simulink model "rocketSim"  (R2020a)
settings: Solver=ode3  StartTime=0.0  StopTime=9.9695  FixedStep=smp.h  MaxStep=simPrm.h  RelTol=1e-3
undefined symbols (not defined in the file): pln, rkt, thr
libraries: sm_lib x6, nesl_utility x6, simulink_extras x2
settings Model: Creator=ggparker  LastModifiedBy=crs20
settings SolverCC: NumberNewtonIterations=4
settings DataIOCC: ReturnWorkspaceOutputs=off  SignalLoggingName=rStates
settings DebuggingCC: PregeneratedLibrarySubsystemCodeDiagnostic=none  ArithmeticOperatorsInVariantConditions=warning
settings SFSimCC: SimUseLocalCustomCode=off  CustomCodeUndefinedFunction=UseInterfaceOnly
settings RTWCC: RTWUseLocalCustomCode=off
settings ExplorerConfigSet: InternalSimMechanicsExplorerSettings="<ExplorerConfiguration><canonicalview>planar_xy</canonicalview><AnimationSetting><BasePlaybackSpeed>1.0</BasePlaybackSpeed><PlaybackSpeedFactor>1.0</PlaybackSpeedFactor></AnimationSetting><TilePanel><TileInfo><Tiles Columns=\"1\" Count=\"1\" Rows=\"1\"><Column Weight=\"1\"/><Row Weight=\"1\"/><Tile Height=\"1\" Width=\"1\" X=\"0\" Y=\"0\"/></Tiles></TileInfo><SceneInfo><SceneViewer><BGColor><R>0.60000002384185791</R><G>0.60000002384185791</G><B>0.60000002384185791</B></BGColor><Camera><DoPerspective>off</DoPerspective><Position><X>282.141547094974555</X><Y>-19.3928666167923893</Y><Z>193.684626557609761</Z></Position><Center><X>282.141547094974555</X><Y>-19.3928666167923893</Y><Z>7.11250308427224809e-07</Z></Center><Up><X>0</X><Y>1</Y><Z>0</Z></Up><ViewLimDist>1</ViewLimDist><YLim>366.074836651506018</YLim><XLim>486.611673109928745</XLim></Camera></SceneViewer></SceneInfo></TilePanel><MechEditorPanel><Cameras/><GfxPanelCameraMap/><VideoCreator><PlaybackSpeedRatio>1.0</PlaybackSpeedRatio><FrameRate>30</FrameRate><VideoFormat>Motion JPEG AVI</VideoFormat><FrameSize>auto</FrameSize></VideoCreator></MechEditorPanel></ExplorerConfiguration>"

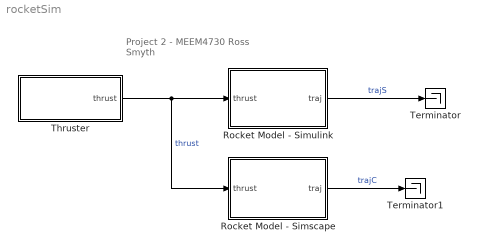
== system rocketSim ==
  note: Project 2 - MEEM4730
      | Ross Smyth
  Rocket Model - Simscape : Subsystem
  Rocket Model - Simulink : Subsystem
  Terminator : Terminator
  Terminator1 : Terminator
  Thruster : Subsystem
  wires:
  Rocket Model - Simulink/1(traj) -> Terminator/1  "trajS"
  Rocket Model - Simscape/1(traj) -> Terminator1/1  "trajC"
  Thruster/1(thrust) -> Rocket Model - Simscape/1(thrust), Rocket Model - Simulink/1(thrust)  "thrust"

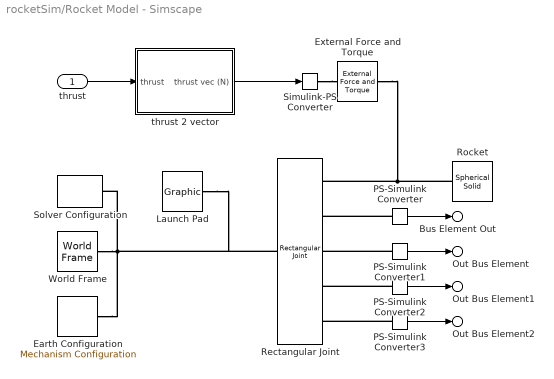
== system rocketSim/Rocket Model - Simscape ==
  thrust : Inport
  Earth Configuration : sm_lib/Utilities/Mechanism Configuration  UniformGravity=Constant  GravityVector=[0 -pln.g 0]  GravityUnits=m/s^2  LinearizationDelta=0.001
  External Force and Torque : sm_lib/Forces and Torques/External Force and Torque  ForceResolutionFrame=AttachedFrame  EnableForceX=off  EnableForceY=off  EnableForceZ=off  EnableForce=on  TorqueResolutionFrame=AttachedFrame  EnableTorqueX=off  EnableTorqueY=off  EnableTorqueZ=off  EnableTorque=off
  Launch Pad : sm_lib/Body Elements/Graphic  GraphicType=Marker  MarkerShape=Cube  MarkerSize=10  GraphicVisPropType=SimpleVisualProperties  GraphicDiffuseColor=[1.0 0.0 0.4]  GraphicSpecularColor=[0.5 0.5 0.5 1.0]  GraphicAmbientColor=[0.15 0.15 0.15 1.0]  GraphicEmissiveColor=[0.0 0.0 0.0 1.0]  GraphicShininess=75  GraphicOpacity=1.0
  PS-Simulink Converter{,1..3} (4 alike) : nesl_utility/PS-Simulink Converter  PhysicalDomain=network_engine_domain  SubClassName=ps_output  LeftPortType=input  RightPortType=output  PseudoPeriodic=off  Frequencies=[]  Unit=inherit  AffineConversion=off
  Rectangular Joint : sm_lib/Joints/Rectangular Joint  JointMode=Normal  SenseConstraintForce=off  SenseConstraintForceX=off  SenseConstraintForceY=off  SenseConstraintForceZ=off  SenseConstraintTorque=off  SenseConstraintTorqueX=off  SenseConstraintTorqueY=off  SenseConstraintTorqueZ=off  SenseTotalForce=off  SenseTotalForceX=off  SenseTotalForceY=off  SenseTotalForceZ=off  SenseTotalTorque=off  SenseTotalTorqueX=off  SenseTotalTorqueY=off  SenseTotalTorqueZ=off  CompositeWrenchDir=FollowerOnBase  CompositeWrenchFrame=BaseFrame  PxEquilibriumPosition=0  PxEquilibriumPositionUnits=m  PxSpringStiffness=0  PxSpringStiffnessUnits=N/m  PxDampingCoefficient=0  PxDampingCoefficientUnits=N/(m/s)  PxTorqueActuationMode=NoTorque  PxMotionActuationMode=ComputedMotion  PxSensePosition=on  PxSenseVelocity=on  PxSenseAcceleration=off  PxSenseTorqueForce=off  PxSenseLowerLimitTorqueForce=off  PxSenseUpperLimitTorqueForce=off  PxLowerLimitSpecify=off  PxLowerLimitBound=0  PxLowerLimitBoundUnits=m  PxLowerLimitStiffness=0  PxLowerLimitStiffnessUnits=N/m  PxLowerLimitDamping=0  PxLowerLimitDampingUnits=N/(m/s)  PxLowerLimitTransitionRegionWidth=0  PxLowerLimitTransitionRegionWidthUnits=m  PxUpperLimitSpecify=off  PxUpperLimitBound=1  PxUpperLimitBoundUnits=m  PxUpperLimitStiffness=1e6  PxUpperLimitStiffnessUnits=N/m  PxUpperLimitDamping=1e3  PxUpperLimitDampingUnits=N/(m/s)  PxUpperLimitTransitionRegionWidth=1e-4  PxUpperLimitTransitionRegionWidthUnits=m  PxPositionTargetSpecify=off  PxPositionTargetPriority=High  PxPositionTargetValue=0  PxPositionTargetValueUnits=m  PxVelocityTargetSpecify=off  PxVelocityTargetPriority=High  PxVelocityTargetValue=0  PxVelocityTargetValueUnits=m/s  PyEquilibriumPosition=0  PyEquilibriumPositionUnits=m  PySpringStiffness=0  PySpringStiffnessUnits=N/m  PyDampingCoefficient=0  PyDampingCoefficientUnits=N/(m/s)  PyTorqueActuationMode=NoTorque  PyMotionActuationMode=ComputedMotion  PySensePosition=on  PySenseVelocity=on  PySenseAcceleration=off  PySenseTorqueForce=off  PySenseLowerLimitTorqueForce=off  PySenseUpperLimitTorqueForce=off  PyLowerLimitSpecify=off  PyLowerLimitBound=-1  PyLowerLimitBoundUnits=m  PyLowerLimitStiffness=1e6  PyLowerLimitStiffnessUnits=N/m  PyLowerLimitDamping=1e3  PyLowerLimitDampingUnits=N/(m/s)  PyLowerLimitTransitionRegionWidth=1e-4  PyLowerLimitTransitionRegionWidthUnits=m  PyUpperLimitSpecify=off  PyUpperLimitBound=1  PyUpperLimitBoundUnits=m  PyUpperLimitStiffness=1e6  PyUpperLimitStiffnessUnits=N/m  PyUpperLimitDamping=1e3  PyUpperLimitDampingUnits=N/(m/s)  PyUpperLimitTransitionRegionWidth=1e-4  PyUpperLimitTransitionRegionWidthUnits=m  PyPositionTargetSpecify=off  PyPositionTargetPriority=High  PyPositionTargetValue=0  PyPositionTargetValueUnits=m  PyVelocityTargetSpecify=off  PyVelocityTargetPriority=High  PyVelocityTargetValue=0  PyVelocityTargetValueUnits=m/s
  Rocket : sm_lib/Body Elements/Spherical Solid  GraphicAmbientColor=[0.15 0.15 0.15 1.0]  BasedOnType=Mass  CenterOfMass=[0 0 0]  CenterOfMassUnits=m  GraphicDiffuseColor=[0.5 0.5 0.5]  Density=rkt.m  DensityUnits=kg/m^3  DoExposeReferenceFrame=on  GraphicEmissiveColor=[0.0 0.0 0.0 1.0]  ExportEntireGeometry=off  SerializedExposedGeometries=<ExposedGeometries/>  SerializedFrames=<Frames/>  MarkerShape=Sphere  MarkerSize=10  GraphicType=FromGeometry  InertiaType=PointMass  Mass=rkt.m  MassUnits=kg  MomentsOfInertia=[1 1 1]  MomentsOfInertiaUnits=kg*m^2  GraphicOpacity=1.0  ProductsOfInertia=[0 0 0]  ProductsOfInertiaUnits=kg*m^2  GraphicShininess=75  GraphicSpecularColor=[0.5 0.5 0.5 1.0]  SphereRadius=1  SphereRadiusUnits=m  GraphicVisPropType=SimpleVisualProperties
  Simulink-PS Converter : nesl_utility/Simulink-PS Converter  PhysicalDomain=network_engine_domain  SubClassName=ps_input  LeftPortType=input  RightPortType=output  PseudoPeriodic=off  Frequencies=[]  NoiseDistribution=none  NoiseParameters=[]  Unit=1  AffineConversion=off  FilteringAndDerivatives=provide  SimscapeFilterOrder=1  InputFilterTimeConstant=0.001  UdotUserProvided=0
  Solver Configuration : nesl_utility/Solver Configuration  PhysicalDomain=network_engine_domain  SubClassName=solver  LeftPortType=input  RightPortType=generic  Tones=[]  Harmonics=[]  SimulateNoise=off  Profile=off  UseLocalSampling=off  EnableSwitchedLinearOptims=on  FrequencyDomain=off  UseCCode=off  RelTol=0.001  AbsTol=1e-06  MinStep=1e-09  ToWorkspace=off  RevertToSquareIcSolve=off  NumHomotopyIterations=100  PhasorMode=off  PhasorModeNumHarmonics=1  DoDC=off  ResidualTolerance=1e-09  UseLocalSolver=off  LocalSolverChoice=NE_BACKWARD_EULER_ADVANCER  LocalSolverSampleTime=0.001  DoFixedCost=off  MaxNonlinIter=3  MaxModeIter=2  LinearAlgebra=auto  EquationFormulation=NE_TIME_EF  DelaysMemoryBudget=1024  AutomaticFiltering=on  FilteringTimeConstant=0.001  PartitionStorageMethod=AS_NEEDED  PartitionMemoryBudget=1024  PartitionMethod=ROBUST
  World Frame : sm_lib/Frames and Transforms/World Frame
  thrust 2 vector : Subsystem
  Bus Element Out : Outport  PortName=traj  Element=x
  Out Bus Element : Outport  PortName=traj  Element=xd
  Out Bus Element1 : Outport  PortName=traj  Element=y
  Out Bus Element2 : Outport  PortName=traj  Element=yd
  wires:
  thrust/1 -> thrust 2 vector/1(thrust)
  thrust 2 vector/1(thrust vec (N)) -> Simulink-PS Converter/1
  PS-Simulink Converter/1 -> Bus Element Out/1
  PS-Simulink Converter1/1 -> Out Bus Element/1
  PS-Simulink Converter2/1 -> Out Bus Element1/1
  PS-Simulink Converter3/1 -> Out Bus Element2/1
  connections:
  World Frame/RConn1 -- Launch Pad/RConn1 -- Rectangular Joint/LConn1 -- Solver Configuration/RConn1 -- Earth Configuration/RConn1
  PS-Simulink Converter/LConn1 -- Rectangular Joint/RConn2
  PS-Simulink Converter1/LConn1 -- Rectangular Joint/RConn3
  PS-Simulink Converter2/LConn1 -- Rectangular Joint/RConn4
  PS-Simulink Converter3/LConn1 -- Rectangular Joint/RConn5
  Simulink-PS Converter/RConn1 -- External Force and Torque/LConn1
  Rocket/RConn1 -- External Force and Torque/RConn1 -- Rectangular Joint/RConn1

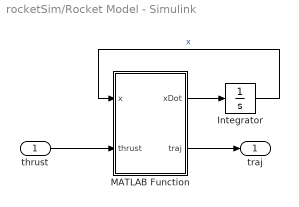
== system rocketSim/Rocket Model - Simulink ==
  thrust : Inport  OutDataTypeStr=Bus: thrust
  Integrator : Integrator  InitialCondition=rkt.ics
  MATLAB Function : MATLAB Function  TreatAsAtomicUnit=on
  traj : Outport  OutDataTypeStr=Bus: traj  VectorParamsAs1DForOutWhenUnconnected=off
  wires:
  MATLAB Function/2(traj) -> traj/1
  thrust/1 -> MATLAB Function/2(thrust)
  MATLAB Function/1(xDot) -> Integrator/1
  Integrator/1 -> MATLAB Function/1(x)  "x"

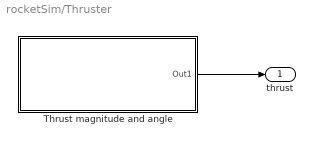
== system rocketSim/Thruster ==
  "Thrust magnitude and angle " : Subsystem  Variant=on  VariantControl=Choice
  thrust : Outport  OutDataTypeStr=Bus: thrust  VectorParamsAs1DForOutWhenUnconnected=off
  wires:
  "Thrust magnitude and angle "/1(Out1) -> thrust/1

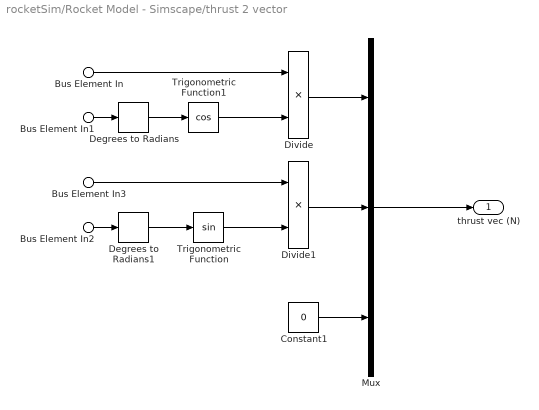
== system rocketSim/Rocket Model - Simscape/thrust 2 vector ==
  Bus Element In : Inport  PortName=thrust  Element=mag
  Bus Element In3 : Inport  PortName=thrust  Element=mag
  Bus Element In1 : Inport  PortName=thrust  Element=ang
  Bus Element In2 : Inport  PortName=thrust  Element=ang
  Constant1 : Constant  Value=0
  Degrees to Radians : simulink_extras/Transformations/Degrees to Radians
  Degrees to Radians1 : simulink_extras/Transformations/Degrees to Radians
  Divide : Product  Inputs=**
  Divide1 : Product  Inputs=**
  Mux : Mux  Inputs=3
  Trigonometric Function : Trigonometry
  Trigonometric Function1 : Trigonometry  Operator=cos
  thrust vec (N) : Outport  VectorParamsAs1DForOutWhenUnconnected=off
  wires:
  Trigonometric Function/1 -> Divide1/2
  Trigonometric Function1/1 -> Divide/2
  Degrees to Radians/1 -> Trigonometric Function1/1
  Bus Element In/1 -> Divide/1
  Bus Element In1/1 -> Degrees to Radians/1
  Bus Element In2/1 -> Degrees to Radians1/1
  Degrees to Radians1/1 -> Trigonometric Function/1
  Bus Element In3/1 -> Divide1/1
  Divide/1 -> Mux/1
  Divide1/1 -> Mux/2
  Constant1/1 -> Mux/3
  Mux/1 -> thrust vec (N)/1

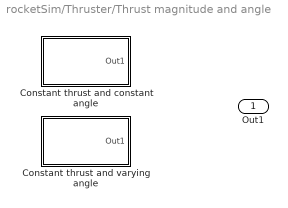
== system rocketSim/Thruster/Thrust magnitude and angle  ==
  Constant thrust and constant angle : Subsystem  VariantControl=SCENARIO==1  mask{magnitude=thr.F, angle=thr.tht, time=rkt.t1}
      mask prompts: magnitude "Magnitude (N)"; angle "Angle (Degrees)"; time "Thrust Time (s)"
  Constant thrust and varying angle : Subsystem  VariantControl=SCENARIO==2  mask{magnitude=thr.F, angle=thr.tht, time=rkt.t1, freq=thr.w, angle_amp=thr.amp}
      mask prompts: magnitude "Thrust Magnitude (N)"; angle "Thrust Average Angle (Degrees)"; time "Thrust Time (s)"; freq "Angle Frequency (rad/s)"; angle_amp "Angle Varying Amplitude (Degrees)"
  Out1 : Outport

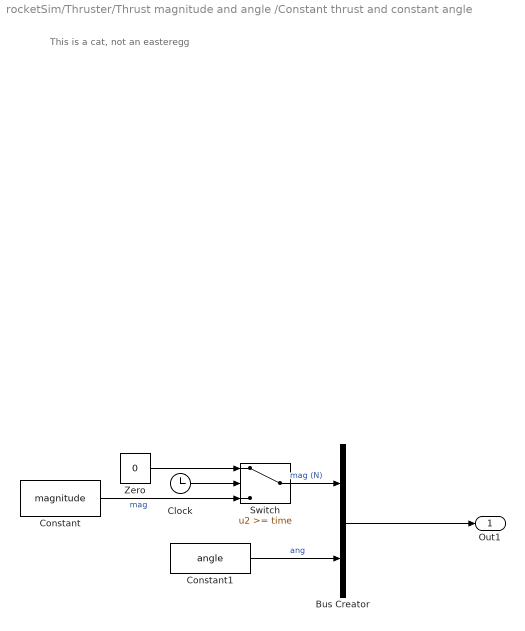
== system rocketSim/Thruster/Thrust magnitude and angle /Constant thrust and constant angle ==
  note: This is a cat, not an easteregg
  Bus Creator : BusCreator  Inputs=2  OutDataTypeStr=Bus: thrust
      settings: InheritFromInputs=off
  Clock : Clock
  Constant : Constant  Value=magnitude
  Constant1 : Constant  Value=angle
  Switch : Switch  Threshold=time
  Zero : Constant  Value=0  OutDataTypeStr=Inherit: Inherit via back propagation
  Out1 : Outport
  wires:
  Constant1/1 -> Bus Creator/2  "ang"
  Bus Creator/1 -> Out1/1
  Constant/1 -> Switch/3  "mag"
  Zero/1 -> Switch/1
  Clock/1 -> Switch/2
  Switch/1 -> Bus Creator/1  "mag (N)"

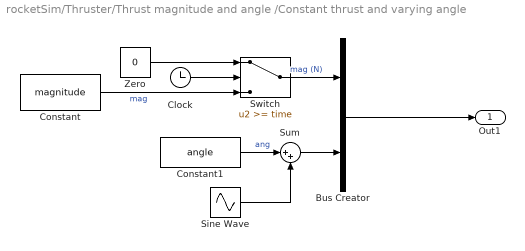
== system rocketSim/Thruster/Thrust magnitude and angle /Constant thrust and varying angle ==
  Bus Creator : BusCreator  Inputs=2  OutDataTypeStr=Bus: thrust
      settings: InheritFromInputs=off
  Clock : Clock
  Constant : Constant  Value=magnitude
  Constant1 : Constant  Value=angle
  Sine Wave : Sin  Amplitude=angle_amp  Frequency=freq  SampleTime=0
  Sum : Sum  Inputs=|++
  Switch : Switch  Threshold=time
  Zero : Constant  Value=0  OutDataTypeStr=Inherit: Inherit via back propagation
  Out1 : Outport
  wires:
  Constant/1 -> Switch/3  "mag"
  Zero/1 -> Switch/1
  Switch/1 -> Bus Creator/1  "mag (N)"
  Bus Creator/1 -> Out1/1
  Clock/1 -> Switch/2
  Sum/1 -> Bus Creator/2
  Constant1/1 -> Sum/1  "ang"
  Sine Wave/1 -> Sum/2

== matlab function rocketSim/Rocket Model - Simulink/MATLAB Function ==
  data: x input; xDot output; thrust input; traj output Bus: traj; pln parameter; rkt parameter
function [xDot, traj] = fcn(x, thrust, pln, rkt)
%   Inputs
%      x = The state(s) of the system at the current time. [1x4 double]
%      thrust = Input thrust bus at current time [thrust]
%      pln    = Planet information struct
%      rkt    = Rocket infomration struct
%
%   Outputs
%       xDot = Derivatives of the states
%       traj = The current states put onto a trajectory bus

% Constants
g = pln.g; % m/s/s
m = rkt.m; % kg

% Initilization
xDot = zeros(4, 1);

% Output
traj.x  = x(1); % m
traj.y  = x(2); % m
traj.xd = x(3); % m/s
traj.yd = x(4); % m/s

xDot(1) = x(3); % m/s
xDot(2) = x(4); % m/s
xDot(3) = thrust.mag/m * cosd(thrust.ang); % m/s/s
xDot(4) = thrust.mag/m * sind(thrust.ang) - g; % m/s/s
